simulink model "simulinkControlLoop"  (R2020b)
settings: Solver=VariableStepAuto  StartTime=0.0  StopTime=11  RelTol=1e-3
undefined symbols (not defined in the file or in its folder): DiscIntNeverNeededParam, equilibrium, K, KI, Kpend, u0jump, u0l, u0r, u3l, u3r
libraries: dspsigops x10, robotgazebolib x5, dspsrcs4 x3, robotcorelib x1
settings Model: Creator=Adam  LastModifiedBy=Adam

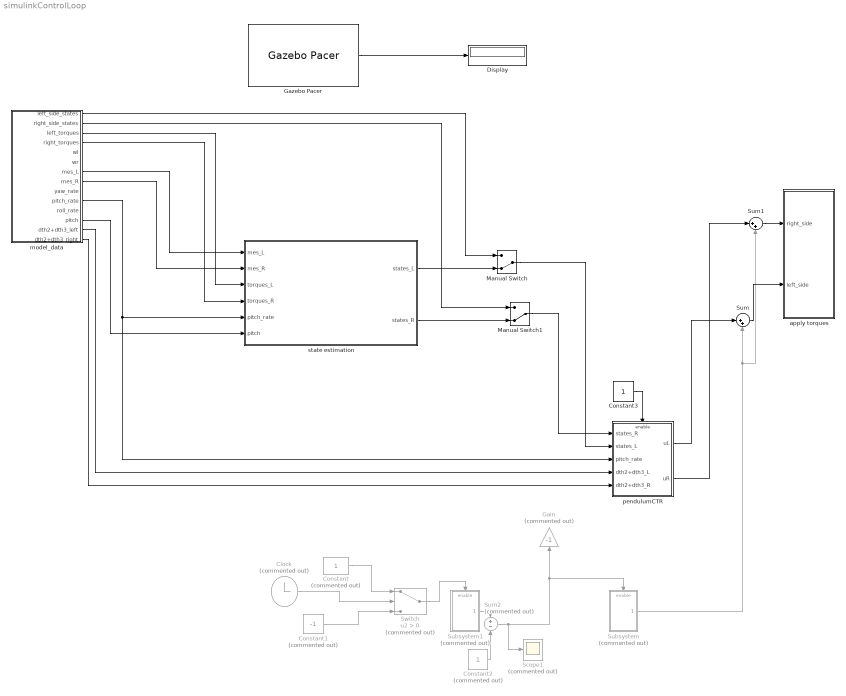
== system simulinkControlLoop ==
  Clock : Clock  Commented=on
  Constant : Constant  Commented=on
  Constant1 : Constant  Commented=on  Value=-1
  Constant2 : Constant  Commented=on
  Constant3 : Constant
  Display : Display
  Gain : Gain  Commented=on  Gain=-1
  Gazebo Pacer : robotgazebolib/Gazebo Pacer  ResetBehavior=Reset Gazebo simulation time and scene  SampleTime=0.001
      settings: SourceProductBaseCode=RO
  Manual Switch : ManualSwitch  CurrentSetting=0
  Manual Switch1 : ManualSwitch  CurrentSetting=0
  Scope1 : Scope  Commented=on
  Subsystem : Subsystem  Commented=on
  Subsystem1 : Subsystem  Commented=on
  Sum : Sum  Inputs=|++
  Sum1 : Sum  Inputs=|++
  Sum2 : Sum  Commented=on  Inputs=+-
  Switch : Switch  Commented=on  Criteria=u2 > Threshold
  apply torques : Subsystem
  model_data : Subsystem
  pendulumCTR : Subsystem
  state estimation : Subsystem
  wires:
  model_data/2(right_side_states) -> Manual Switch1/1
  Manual Switch/1 -> pendulumCTR/2(states_L)
  model_data/1(left_side_states) -> Manual Switch/1
  Manual Switch1/1 -> pendulumCTR/1(states_R)
  Gazebo Pacer/1 -> Display/1
  Constant/1 -> Switch/1
  Constant1/1 -> Switch/3
  Subsystem1/1(Output) -> Sum2/1
  Constant2/1 -> Sum2/2
  Sum2/1 -> Scope1/1, Subsystem/Enable, Gain/1
  Subsystem/1(Output) -> Sum1/2, Sum/2
  Sum1/1 -> apply torques/1(right_side)
  Sum/1 -> apply torques/2(left_side)
  pendulumCTR/1(uL) -> Sum/1
  pendulumCTR/2(uR) -> Sum1/1
  Clock/1 -> Switch/2
  Switch/1 -> Subsystem1/Enable
  Constant3/1 -> pendulumCTR/Enable
  model_data/3(left_torques) -> state estimation/3(torques_L)
  model_data/4(right_torques) -> state estimation/4(torques_R)
  state estimation/1(states_L) -> Manual Switch/2
  state estimation/2(states_R) -> Manual Switch1/2
  model_data/12(pitch) -> state estimation/6(pitch)
  model_data/7(mes_L) -> state estimation/1(mes_L)
  model_data/8(mes_R) -> state estimation/2(mes_R)
  model_data/10(pitch_rate) -> pendulumCTR/3(pitch_rate), state estimation/5(pitch_rate)
  model_data/13(dth2+dth3_left) -> pendulumCTR/4(dth2+dth3_L)
  model_data/14(dth2+dth3_right) -> pendulumCTR/5(dth2+dth3_R)

== system simulinkControlLoop/Subsystem ==
  Enable : EnablePort  StatesWhenEnabling=reset
  Mux : Mux  Inputs=2
  Signal From Workspace : dspsrcs4/Signal From Workspace  X=u3jump  Ts=0.001  nsamps=1  OutputAfterFinalValue=Setting to zero  ignoreOrWarnInputAndFrameLengths=off  OutputFrames=off
  Signal From Workspace1 : dspsrcs4/Signal From Workspace  X=u0jump  Ts=0.001  nsamps=1  OutputAfterFinalValue=Setting to zero  ignoreOrWarnInputAndFrameLengths=off  OutputFrames=off
  Output : Outport
  wires:
  Signal From Workspace1/1 -> Mux/1
  Signal From Workspace/1 -> Mux/2
  Mux/1 -> Output/1

== system simulinkControlLoop/Subsystem1 ==
  Enable : EnablePort  StatesWhenEnabling=reset
  Signal From Workspace : dspsrcs4/Signal From Workspace  X=2*ones(numel(u0jump),1)  Ts=0.001  nsamps=1  OutputAfterFinalValue=Setting to zero  ignoreOrWarnInputAndFrameLengths=off  OutputFrames=off
  Output : Outport
  wires:
  Signal From Workspace/1 -> Output/1

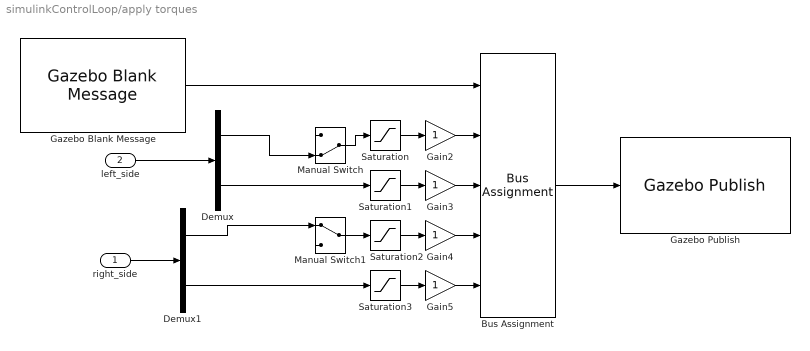
== system simulinkControlLoop/apply torques ==
  right_side : Inport
  left_side : Inport  Port=2
  Bus Assignment : BusAssignment  AssignedSignals=u0l,u3l,u0r,u3r
  Demux : Demux  Outputs=2
  Demux1 : Demux  Outputs=2
  Gain{2..5} (4 alike) : Gain
  Gazebo Blank Message : robotgazebolib/Gazebo Blank Message  msgType=gazebo_msgs/custom/19XzAhyZzP/Contro1XtejReiyv  sampleTime=0.001  busName='Gazebo_SL_Bus_gazebo_msgs_custom_19XzAhyZzP_Contro1XtejReiyv'
      settings: SourceProductBaseCode=RO
  Gazebo Publish : robotgazebolib/Gazebo Publish  topicSource=Specify your own  topic=/gazebo/default/controlCommand  messageType=gazebo_msgs/custom/19XzAhyZzP/Contro1XtejReiyv  sampleTime=0.001
      settings: SourceProductBaseCode=RO
  Manual Switch : ManualSwitch  CurrentSetting=0
  Manual Switch1 : ManualSwitch
  Saturation : Saturate  UpperLimit=2  LowerLimit=-2
  Saturation1 : Saturate  UpperLimit=10  LowerLimit=-10
  Saturation2 : Saturate  UpperLimit=2  LowerLimit=-2
  Saturation3 : Saturate  UpperLimit=10  LowerLimit=-10
  wires:
  Gain3/1 -> Bus Assignment/3
  Saturation3/1 -> Gain5/1
  Saturation/1 -> Gain2/1
  Demux/2 -> Saturation1/1
  Bus Assignment/1 -> Gazebo Publish/1
  Saturation1/1 -> Gain3/1
  Demux1/2 -> Saturation3/1
  Gazebo Blank Message/1 -> Bus Assignment/1
  Gain5/1 -> Bus Assignment/5
  Saturation2/1 -> Gain4/1
  left_side/1 -> Demux/1
  right_side/1 -> Demux1/1
  Demux1/1 -> Manual Switch1/1
  Demux/1 -> Manual Switch/2
  Gain2/1 -> Bus Assignment/2
  Gain4/1 -> Bus Assignment/4
  Manual Switch/1 -> Saturation/1
  Manual Switch1/1 -> Saturation2/1

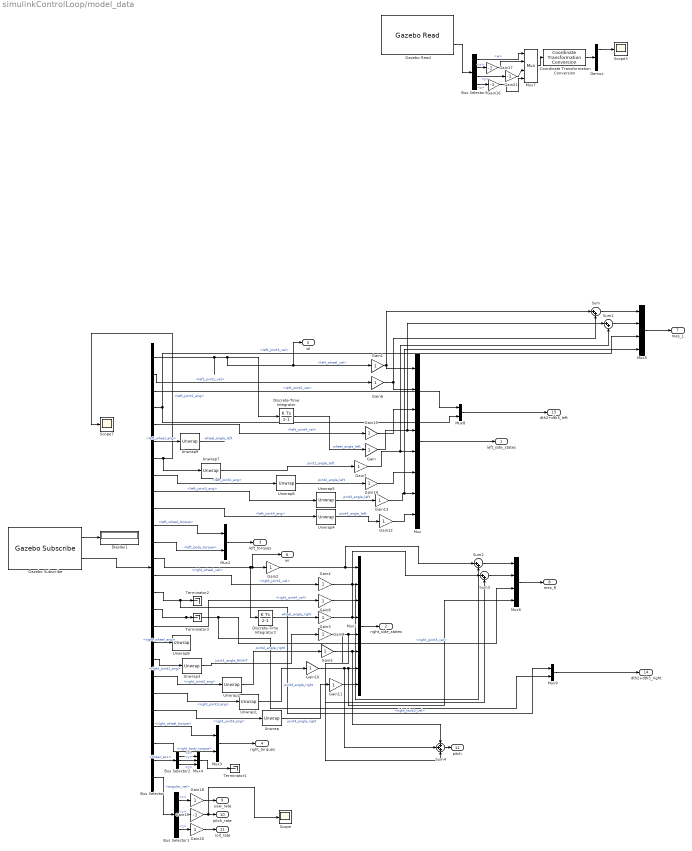
== system simulinkControlLoop/model_data ==
  Bus Selector : BusSelector  OutputSignals=left_wheel_vel,left_joint1_vel,left_joint2_vel,left_joint3_vel,left_joint4_vel,left_wheel_ang,left_joint1_ang,left_joint2_ang,left_joint3_ang,left_joint4_ang,left_wheel_torque,left_body_torque,right_wheel_vel,right_joint1_vel,right_joint2_vel,right_joint3_vel,right_joint4_vel,right_wheel_ang,right_joint1_ang,right_joint2_ang,right_joint3_ang,right_joint4_ang,right_wheel_torque,right_body_torque,linear_acc,angular_vel
  Bus Selector1 : BusSelector  OutputSignals=x,y,z
  Bus Selector2 : BusSelector  OutputSignals=x,y,z
  Bus Selector3 : BusSelector  OutputSignals=world_pose.orientation.w,world_pose.orientation.x,world_pose.orientation.y,world_pose.orientation.z
  Coordinate Transformation Conversion : robotcorelib/Coordinate Transformation Conversion  InputRepresentation=Quaternion  InputEulerSequence=ZYX  ShowTrVecInputPort=on  OutputRepresentation=Euler Angles  OutputEulerSequence=ZYX  ShowTrVecOutputPort=on  SimulateUsing=Interpreted execution
  Demux : Demux  Outputs=3
  Discrete-Time Integrator : DiscreteIntegrator  gainval=1  SampleTime=-1  ICPrevOutput=DiscIntNeverNeededParam  ICPrevScaledInput=DiscIntNeverNeededParam
  Discrete-Time Integrator2 : DiscreteIntegrator  gainval=1  SampleTime=-1  ICPrevOutput=DiscIntNeverNeededParam  ICPrevScaledInput=DiscIntNeverNeededParam
  Display1 : Display
  Gain{,1..15,18,20} (18 alike) : Gain
  Gain{16..17,19,21} (4 alike) : Gain  Gain=-1
  Gazebo Read : robotgazebolib/Gazebo Read  topicSource=From Gazebo  topic=/gazebo/ground_truth/link_state/Stoupento/Stoupento::left_wheel  messageType=gazebo_msgs/LinkState  sampleTime=0.001
      settings: SourceProductBaseCode=RO
  Gazebo Subscribe : robotgazebolib/Gazebo Subscribe  topicSource=From Gazebo  topic=/gazebo/default/stoupentoMesurement  messageType=gazebo_msgs/custom/19XzAhyZzP/Stoupe1grC5VeUzD  sampleTime=0.001
      settings: SourceProductBaseCode=RO
  Mux : Mux  Inputs=8
  Mux1 : Mux  Inputs=8
  Mux{2..3,8..9} (4 alike) : Mux  Inputs=2
  Mux4 : Mux  Inputs=3
  Mux5 : Mux
  Mux6 : Mux
  Mux7 : Mux
  Scope : Scope
  Scope3 : Scope
  Scope7 : Scope
  Sum{,1..3} (4 alike) : Sum  Inputs=|++
  Sum4 : Sum  Inputs=+++
  Terminator1 : Terminator
  Terminator2 : Terminator
  Terminator3 : Terminator
  Unwrap{,1..2,4..6} (6 alike) : dspsigops/Unwrap  tol=pi  InputProcessing=Columns as channels (frame based)  running=off
  Unwrap3 : dspsigops/Unwrap  tol=19/10*pi  InputProcessing=Columns as channels (frame based)  running=off
  Unwrap7 : dspsigops/Unwrap  tol=19/10*pi  InputProcessing=Columns as channels (frame based)  running=off
  Unwrap8 : dspsigops/Unwrap  tol=19*pi/10  InputProcessing=Columns as channels (frame based)  running=off
  Unwrap9 : dspsigops/Unwrap  tol=19/10*pi  InputProcessing=Columns as channels (frame based)  running=off
  left_side_states : Outport
  right_side_states : Outport  Port=2
  left_torques : Outport  Port=3
  right_torques : Outport  Port=4
  wl : Outport  Port=5
  wr : Outport  Port=6
  mes_L : Outport  Port=7
  mes_R : Outport  Port=8
  yaw_rate : Outport  Port=9
  pitch_rate : Outport  Port=10
  roll_rate : Outport  Port=11
  pitch : Outport  Port=12
  dth2+dth3_left : Outport  Port=13
  dth2+dth3_right : Outport  Port=14
  wires:
  Gazebo Subscribe/1 -> Display1/1
  Bus Selector/23 -> Mux3/1  "<right_wheel_torque>"
  Bus Selector/12 -> Mux2/2  "<left_body_torque>"
  Bus Selector/18 -> Unwrap8/1  "<right_wheel_ang>"
  Bus Selector/5 -> Gain15/1  "<left_joint4_vel>"
  Bus Selector/9 -> Unwrap5/1  "<left_joint3_ang>"
  Bus Selector/20 -> Unwrap2/1  "<right_joint2_ang>"
  Bus Selector/22 -> Unwrap/1  "<right_joint4_ang>"
  Bus Selector/8 -> Unwrap6/1  "<left_joint2_ang>"
  Unwrap1/1 -> Gain10/1  "joint3_angle_right"
  Unwrap/1 -> Gain11/1  "joint4_angle_right"
  Unwrap4/1 -> Gain12/1  "joint4_angle_left"
  Gazebo Subscribe/2 -> Bus Selector/1
  Bus Selector/19 -> Unwrap3/1  "<right_joint1_ang>"
  Bus Selector/6 -> Unwrap9/1  "<left_wheel_ang>"
  Unwrap5/1 -> Gain13/1  "joint3_angle_left"
  Bus Selector/7 -> Unwrap7/1, Scope7/1  "<left_joint1_ang>"
  Bus Selector/10 -> Unwrap4/1  "<left_joint4_ang>"
  Unwrap6/1 -> Gain14/1  "joint2_angle_left"
  Bus Selector/21 -> Unwrap1/1  "<right_joint3_ang>"
  Unwrap9/1 -> ?  "wheel_angle_left"
  Mux/1 -> left_side_states/1
  Bus Selector/24 -> Mux3/2  "<right_body_torque>"
  Bus Selector/3 -> Mux8/1  "<left_joint2_vel>"
  Bus Selector/11 -> Mux2/1  "<left_wheel_torque>"
  Mux2/1 -> left_torques/1
  Mux3/1 -> right_torques/1
  Bus Selector/17 -> Gain8/1  "<right_joint4_vel>"
  Bus Selector/13 -> Discrete-Time Integrator2/1, wr/1, Gain2/1  "<right_wheel_vel>"
  Unwrap2/1 -> Gain5/1  "joint2_angle_right"
  Mux1/1 -> right_side_states/1
  Gain3/1 -> Sum3/1, Mux1/4
  Gain4/1 -> Sum2/2, Mux1/2
  Gain5/1 -> Sum4/1, Mux1/6
  Gain8/1 -> Mux1/3
  Gain11/1 -> Mux1/8
  Bus Selector/25 -> Bus Selector2/1  "<linear_acc>"
  Bus Selector/4 -> Mux5/3, Mux8/2  "<left_joint3_vel>"
  Bus Selector/26 -> Bus Selector1/1  "<angular_vel>"
  Gain10/1 -> Sum4/2, Mux6/4, Mux1/7
  Bus Selector2/1 -> Mux4/1  "<x>"
  Bus Selector2/2 -> Mux4/2  "<y>"
  Bus Selector2/3 -> Mux4/3  "<z>"
  Gain2/1 -> Sum2/1, Mux1/1
  Bus Selector/1 -> Discrete-Time Integrator/1, Gain1/1, wl/1  "<left_wheel_vel>"
  Gain1/1 -> Sum/1, Mux/1
  Gain6/1 -> Sum/2, Mux/2
  Mux5/1 -> mes_L/1
  Mux6/1 -> mes_R/1
  Mux4/1 -> Terminator1/1
  Bus Selector1/1 -> Gain18/1  "<x>"
  Bus Selector1/2 -> Gain19/1  "<y>"
  Bus Selector1/3 -> Gain20/1  "<z>"
  Gain18/1 -> yaw_rate/1
  Gain19/1 -> Scope/1, pitch_rate/1
  Gain20/1 -> roll_rate/1
  Gazebo Read/2 -> Bus Selector3/1
  Bus Selector3/1 -> Mux7/1  "<w>"
  Bus Selector3/2 -> Gain17/1  "<x>"
  Bus Selector3/3 -> Gain21/1  "<y>"
  Bus Selector3/4 -> Gain16/1  "<z>"
  Mux7/1 -> Coordinate Transformation Conversion/1
  Coordinate Transformation Conversion/1 -> Demux/1
  Gain16/1 -> Mux7/4
  Gain21/1 -> Mux7/3
  Gain17/1 -> Mux7/2
  Demux/1 -> Scope3/1
  Discrete-Time Integrator/1 -> Gain/1  "wheel_angle_left"
  Discrete-Time Integrator2/1 -> Gain3/1  "wheel_angle_right"
  Bus Selector/2 -> Gain6/1  "<left_joint1_vel>"
  Bus Selector/14 -> Gain4/1  "<right_joint1_vel>"
  Unwrap3/1 -> Gain9/1  "joint1_angle_RIGHT"
  Unwrap7/1 -> Gain7/1  "joint1_angle_left"
  Sum/1 -> Mux5/1
  Sum1/1 -> Mux5/2
  Sum2/1 -> Mux6/1
  Sum3/1 -> Mux6/2
  Gain9/1 -> Sum3/2, Sum4/3, Mux1/5
  Sum4/1 -> pitch/1
  Gain15/1 -> Mux/3
  Gain/1 -> Sum1/1, Mux/4
  Gain7/1 -> Sum1/2, Mux/5
  Gain14/1 -> Mux/6
  Gain13/1 -> Mux5/4, Mux/7
  Gain12/1 -> Mux/8
  Mux8/1 -> dth2+dth3_left/1
  Bus Selector/16 -> Mux9/2, Mux6/3, Terminator3/1  "<right_joint3_vel>"
  Mux9/1 -> dth2+dth3_right/1
  Bus Selector/15 -> Mux9/1, Terminator2/1  "<right_joint2_vel>"

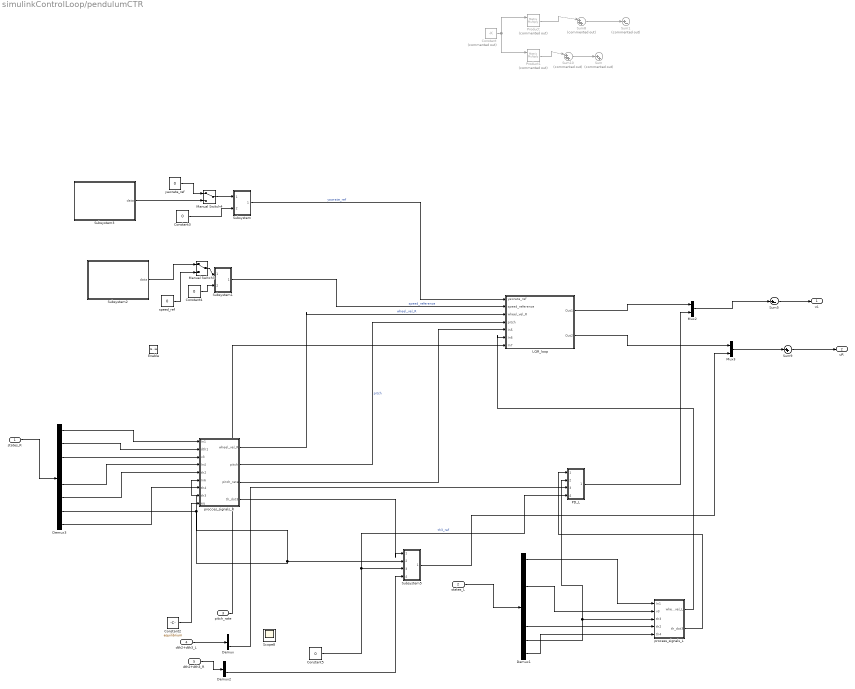
== system simulinkControlLoop/pendulumCTR ==
  states_R : Inport
  states_L : Inport  Port=2
  pitch_rate : Inport  Port=3
  dth2+dth3_L : Inport  Port=4
  dth2+dth3_R : Inport  Port=5
  Enable : EnablePort  StatesWhenEnabling=reset
  Constant : Constant  Commented=on  Value=-K
  Constant2 : Constant  Value=equilibrium
  Constant3 : Constant  Value=0
  Constant4 : Constant  Value=0
  Constant5 : Constant  Value=0
  Demux : Demux  Outputs=2
  Demux1 : Demux  Outputs=8
  Demux2 : Demux  Outputs=2
  Demux3 : Demux  Outputs=8
  LQR_loop : Subsystem
  Manual Switch3 : ManualSwitch
  Manual Switch4 : ManualSwitch
  Mux2 : Mux  Inputs=2
  Mux3 : Mux  Inputs=3
  PD_L : Subsystem
  Product : Product  Commented=on  Multiplication=Matrix(*)
  Product1 : Product  Commented=on  Multiplication=Matrix(*)
  Scope8 : Scope  NumInputPorts=2
  Subsystem : Subsystem
  Subsystem1 : Subsystem
  Subsystem2 : Subsystem
  Subsystem3 : Subsystem
  Subsystem5 : Subsystem
  Sum : Sum  Commented=on  Inputs=|++
  Sum1 : Sum  Commented=on  Inputs=|+-
  Sum10 : Sum  Commented=on  Inputs=|+++
  Sum5 : Sum  Inputs=|+-
  Sum8 : Sum  Commented=on  Inputs=|+++
  Sum9 : Sum  Inputs=|++
  procces_signals_R : Subsystem
  process_signals_L : Subsystem
  speed_ref : Constant  Value=0  SampleTime=0.001
  yawrate_ref : Constant  Value=0  SampleTime=0.001
  uL : Outport
  uR : Outport  Port=2
  wires:
  Constant/1 -> Product/1, Product1/1
  Product/1 -> Sum8/1
  Sum8/1 -> Sum1/1
  Product1/1 -> Sum10/1
  Sum10/1 -> Sum/1
  states_R/1 -> Demux3/1
  states_L/1 -> Demux1/1
  Demux3/7 -> procces_signals_R/8(th3), Subsystem5/2(In2), procces_signals_R/6(In6)
  Sum5/1 -> uL/1
  Mux2/1 -> Sum5/1
  Sum9/1 -> uR/1
  Mux3/1 -> Sum9/1
  Constant3/1 -> Subsystem/2(lambda)
  Constant4/1 -> Subsystem1/2(lambda)
  Constant5/1 -> PD_L/4(th3_ref), Subsystem5/3(th3_ref)  "th3_ref"
  Demux1/7 -> process_signals_L/3(th3), PD_L/2(In2)
  dth2+dth3_L/1 -> Demux/1
  dth2+dth3_R/1 -> Demux2/1
  Subsystem2/1(data) -> Manual Switch3/1
  Manual Switch4/1 -> Subsystem/1(data)
  Subsystem3/1(data) -> Manual Switch4/2
  yawrate_ref/1 -> Manual Switch4/1
  Manual Switch3/1 -> Subsystem1/1(data)
  speed_ref/1 -> Manual Switch3/2
  Demux3/1 -> procces_signals_R/1(In1)
  Demux3/2 -> procces_signals_R/2(dth1)
  Demux3/3 -> procces_signals_R/3(v3)
  Demux3/5 -> procces_signals_R/4(In4)
  Demux3/6 -> procces_signals_R/5(th2)
  Demux3/8 -> procces_signals_R/7(th4)
  Constant2/1 -> procces_signals_R/9(eq)
  procces_signals_R/4(th_dot3) -> Subsystem5/1(In1)
  Demux2/2 -> Subsystem5/4(In4)
  Subsystem5/1(Out1) -> Mux3/3
  Demux/2 -> PD_L/3(In3)
  PD_L/1(Out1) -> Mux2/2
  Demux1/1 -> process_signals_L/1(In1)
  Demux1/3 -> process_signals_L/2(v3)
  Demux1/6 -> process_signals_L/4(th2)
  Demux1/8 -> process_signals_L/5(th4)
  process_signals_L/2(th_dot3) -> PD_L/1(In1)
  Subsystem/1(Out1) -> LQR_loop/1(yawrate_ref)  "yawrate_ref"
  Subsystem1/1(Out1) -> LQR_loop/2(speed_reference)  "speed_reference"
  procces_signals_R/1(wheel_vel_R) -> LQR_loop/3(wheel_vel_R)  "wheel_vel_R"
  procces_signals_R/2(pitch) -> LQR_loop/4(pitch)  "pitch"
  procces_signals_R/3(pitch_rate) -> LQR_loop/5(In5)
  process_signals_L/1(wheel_vel_L) -> LQR_loop/6(In6)
  pitch_rate/1 -> LQR_loop/7(In7)
  LQR_loop/1(Out1) -> Mux2/1
  LQR_loop/2(Out2) -> Mux3/1

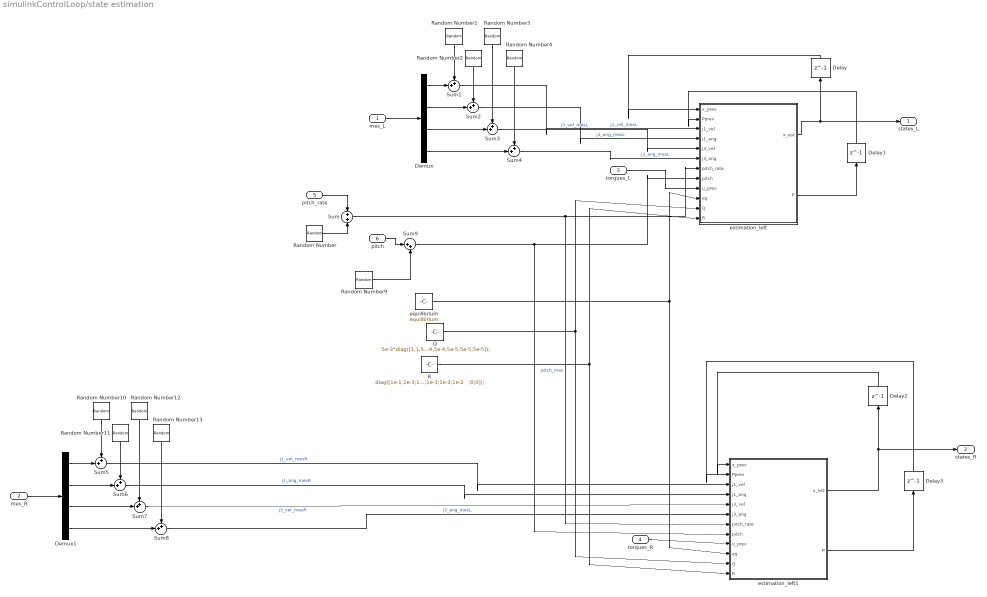
== system simulinkControlLoop/state estimation ==
  mes_L : Inport
  mes_R : Inport  Port=2
  torques_L : Inport  Port=3
  torques_R : Inport  Port=4
  pitch_rate : Inport  Port=5
  pitch : Inport  Port=6
  Delay : Delay  DelayLength=1  InitialCondition=[0;0;0;0;0;0;0;0]  SampleTime=0.001
  Delay1 : Delay  DelayLength=1  InitialCondition=1e-6*eye(8)  SampleTime=0.001
  Delay2 : Delay  DelayLength=1  InitialCondition=[0;0;0;0;0;0;0;0]  SampleTime=0.001
  Delay3 : Delay  DelayLength=1  InitialCondition=1e-6*eye(8)  SampleTime=0.001
  Demux : Demux
  Demux1 : Demux
  Q : Constant  Value=5e-3*diag([1,1,5e-2,5e-4,5e-4,5e-5,5e-5,5e-5]);
  R : Constant  Value="diag([1e-1;1e-3;1e-1;1e-3;1e-2;1e-2   ;0;0]);"
  Random Number : RandomNumber  Variance=1e-2  Seed=randi([0 100])  SampleTime=0.001
  Random Number{1,3,10,12} (4 alike) : RandomNumber  Variance=1e-1  Seed=randi([0 100])  SampleTime=0.001
  Random Number{2,4,11,13} (4 alike) : RandomNumber  Variance=1e-3  Seed=randi([0 100])  SampleTime=0.001
  Random Number9 : RandomNumber  Variance=1e-2  Seed=randi([0 100])  SampleTime=0.001
  Sum : Sum
  Sum{1..8} (8 alike) : Sum  Inputs=++|
  Sum9 : Sum  Inputs=|++
  equilibrium : Constant  Value=equilibrium
  estimation_left : MATLAB Function  TreatAsAtomicUnit=on
  estimation_left1 : MATLAB Function  TreatAsAtomicUnit=on
  states_L : Outport
  states_R : Outport  Port=2
  wires:
  torques_L/1 -> estimation_left/9(u_prev)
  estimation_left/1(x_est) -> states_L/1, Delay/1
  Delay/1 -> estimation_left/1(x_prev)
  estimation_left/2(P) -> Delay1/1
  Delay1/1 -> estimation_left/2(Pprev)
  pitch_rate/1 -> Sum/1
  Random Number/1 -> Sum/2
  mes_L/1 -> Demux/1
  Demux/1 -> Sum1/2
  Demux/2 -> Sum2/2
  Demux/3 -> Sum3/2
  Demux/4 -> Sum4/2
  Random Number4/1 -> Sum4/1
  Random Number3/1 -> Sum3/1
  Random Number2/1 -> Sum2/1
  Random Number1/1 -> Sum1/1
  Sum1/1 -> estimation_left/3(j1_vel)  "j1_vel_mesL"
  Sum2/1 -> estimation_left/4(j1_ang)  "j1_ang_mesL"
  Sum3/1 -> estimation_left/5(j3_vel)  "j3_vel_mesL"
  Sum4/1 -> estimation_left/6(j3_ang)  "j3_ang_mesL"
  R/1 -> estimation_left1/12(R), estimation_left/12(R)
  Sum/1 -> estimation_left1/7(pitch_rate), estimation_left/7(pitch_rate)  "pitch_mes"
  Sum5/1 -> estimation_left1/3(j1_vel)  "j1_vel_mesR"
  Sum8/1 -> estimation_left1/6(j3_ang)  "j3_ang_mesL"
  Sum6/1 -> estimation_left1/4(j1_ang)  "j1_ang_mesR"
  Random Number13/1 -> Sum8/1
  Random Number11/1 -> Sum6/1
  equilibrium/1 -> estimation_left1/10(eq), estimation_left/10(eq)
  Demux1/4 -> Sum8/2
  Q/1 -> estimation_left/11(Q), estimation_left1/11(Q)
  Sum7/1 -> estimation_left1/5(j3_vel)  "j3_vel_mesR"
  Demux1/2 -> Sum6/2
  torques_R/1 -> estimation_left1/9(u_prev)
  mes_R/1 -> Demux1/1
  Demux1/3 -> Sum7/2
  Demux1/1 -> Sum5/2
  pitch/1 -> Sum9/1
  Random Number9/1 -> Sum9/2
  Sum9/1 -> estimation_left1/8(pitch), estimation_left/8(pitch)
  Random Number10/1 -> Sum5/1
  Random Number12/1 -> Sum7/1
  estimation_left1/2(P) -> Delay3/1
  Delay2/1 -> estimation_left1/1(x_prev)
  estimation_left1/1(x_est) -> states_R/1, Delay2/1
  Delay3/1 -> estimation_left1/2(Pprev)

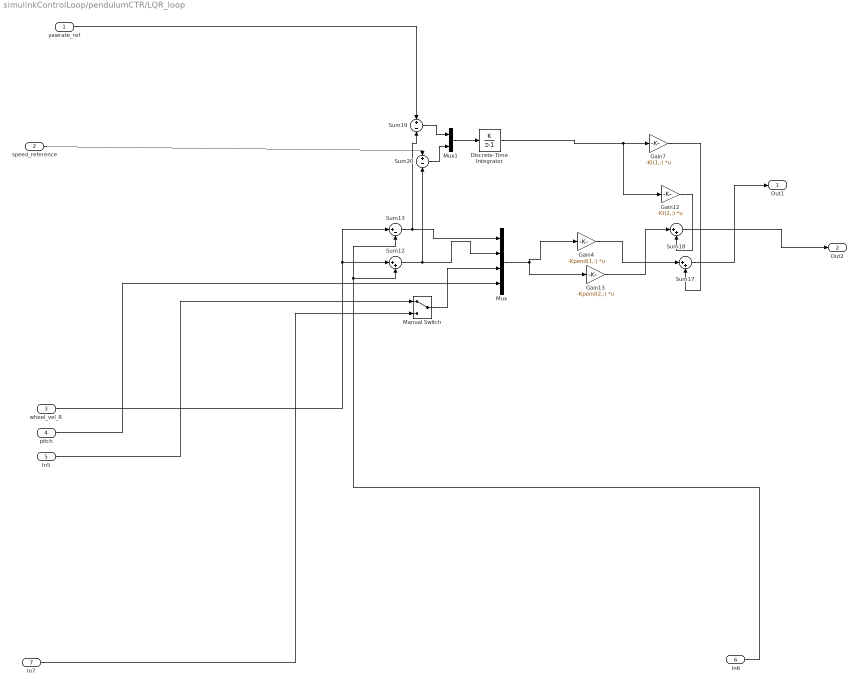
== system simulinkControlLoop/pendulumCTR/LQR_loop ==
  yawrate_ref : Inport
  speed_reference : Inport  Port=2
  wheel_vel_R : Inport  Port=3
  pitch : Inport  Port=4
  In5 : Inport  Port=5
  In6 : Inport  Port=6
  In7 : Inport  Port=7
  Discrete-Time Integrator : DiscreteIntegrator  IntegratorMethod=Accumulation: Forward Euler  gainval=1  SampleTime=0.001  ICPrevOutput=DiscIntNeverNeededParam  ICPrevScaledInput=DiscIntNeverNeededParam
  Gain12 : Gain  Gain=-KI(2,:)  Multiplication=Matrix(K*u)
  Gain13 : Gain  Gain=-Kpend(2,:)  Multiplication=Matrix(K*u)
  Gain4 : Gain  Gain=-Kpend(1,:)  Multiplication=Matrix(K*u)
  Gain7 : Gain  Gain=-KI(1,:)  Multiplication=Matrix(K*u)
  Manual Switch : ManualSwitch
  Mux : Mux
  Mux1 : Mux  Inputs=2
  Sum12 : Sum  Inputs=|++
  Sum13 : Sum  Inputs=|+-
  Sum17 : Sum  Inputs=|++
  Sum18 : Sum  Inputs=|++
  Sum19 : Sum  Inputs=+-
  Sum20 : Sum  Inputs=+-
  Out1 : Outport
  Out2 : Outport  Port=2
  wires:
  Discrete-Time Integrator/1 -> Gain12/1, Gain7/1
  wheel_vel_R/1 -> Sum13/1, Sum12/1
  Sum13/1 -> Sum19/2, Mux/1
  yawrate_ref/1 -> Sum19/1
  Sum19/1 -> Mux1/1
  Sum12/1 -> Sum20/2, Mux/2
  Mux/1 -> Gain4/1, Gain13/1
  In6/1 -> Sum12/2, Sum13/2
  Gain12/1 -> Sum18/2
  Gain4/1 -> Sum17/1
  Mux1/1 -> Discrete-Time Integrator/1
  Sum20/1 -> Mux1/2
  pitch/1 -> Mux/4
  Manual Switch/1 -> Mux/3
  Gain13/1 -> Sum18/1
  Gain7/1 -> Sum17/2
  Sum17/1 -> Out1/1
  Sum18/1 -> Out2/1
  In7/1 -> Manual Switch/2
  speed_reference/1 -> Sum20/1
  In5/1 -> Manual Switch/1

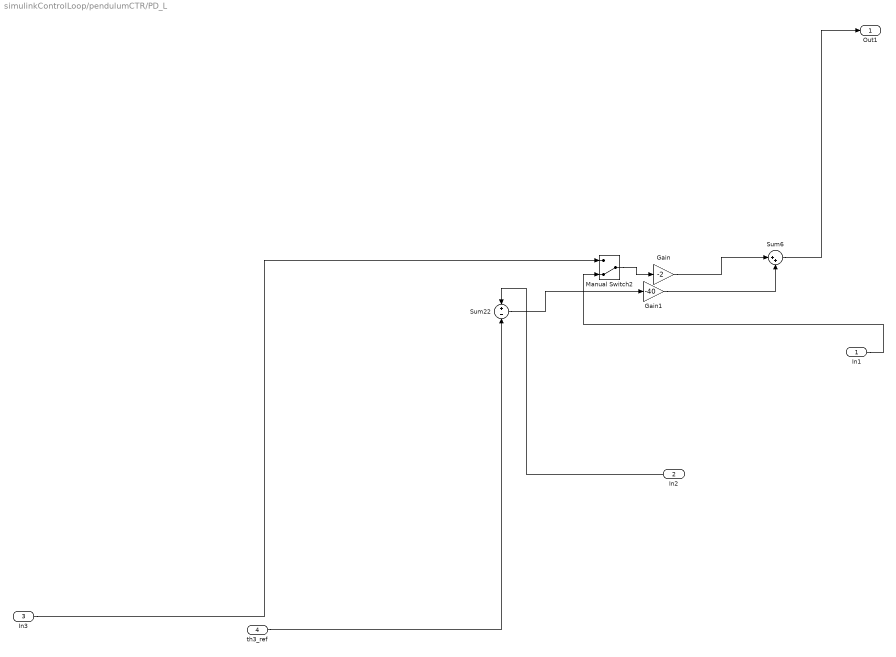
== system simulinkControlLoop/pendulumCTR/PD_L ==
  In1 : Inport
  In2 : Inport  Port=2
  In3 : Inport  Port=3
  th3_ref : Inport  Port=4
  Gain : Gain  Gain=-2
  Gain1 : Gain  Gain=-40
  Manual Switch2 : ManualSwitch  CurrentSetting=0
  Sum22 : Sum  Inputs=+-
  Sum6 : Sum  Inputs=|++
  Out1 : Outport
  wires:
  In3/1 -> Manual Switch2/1
  In2/1 -> Sum22/1
  th3_ref/1 -> Sum22/2
  Gain1/1 -> Sum6/2
  Gain/1 -> Sum6/1
  Sum22/1 -> Gain1/1
  Sum6/1 -> Out1/1
  In1/1 -> Manual Switch2/2
  Manual Switch2/1 -> Gain/1

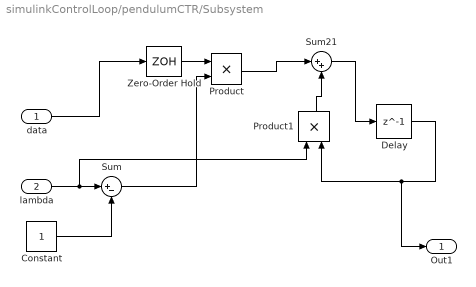
== system simulinkControlLoop/pendulumCTR/Subsystem ==
  data : Inport
  lambda : Inport  Port=2
  Constant : Constant
  Delay : Delay  DelayLength=1  SampleTime=0.01
  Product : Product
  Product1 : Product
  Sum : Sum  Inputs=|+-
  Sum21 : Sum  Inputs=|++
  Zero-Order Hold : ZeroOrderHold  SampleTime=0.01
  Out1 : Outport
  wires:
  Sum21/1 -> Delay/1
  Delay/1 -> Product1/2, Out1/1
  Product/1 -> Sum21/1
  Zero-Order Hold/1 -> Product/1
  lambda/1 -> Product1/1, Sum/1
  Constant/1 -> Sum/2
  Sum/1 -> Product/2
  Product1/1 -> Sum21/2
  data/1 -> Zero-Order Hold/1

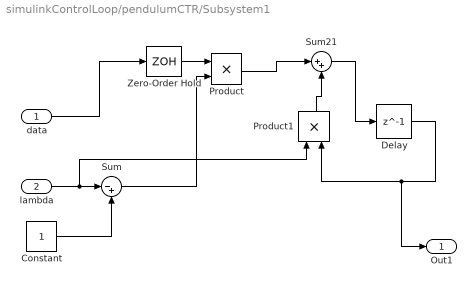
== system simulinkControlLoop/pendulumCTR/Subsystem1 ==
  data : Inport
  lambda : Inport  Port=2
  Constant : Constant
  Delay : Delay  DelayLength=1  SampleTime=0.01
  Product : Product
  Product1 : Product
  Sum : Sum  Inputs=|-+
  Sum21 : Sum  Inputs=|++
  Zero-Order Hold : ZeroOrderHold  SampleTime=0.01
  Out1 : Outport
  wires:
  Sum21/1 -> Delay/1
  Delay/1 -> Product1/2, Out1/1
  Product/1 -> Sum21/1
  Zero-Order Hold/1 -> Product/1
  lambda/1 -> Product1/1, Sum/1
  Constant/1 -> Sum/2
  Sum/1 -> Product/2
  Product1/1 -> Sum21/2
  data/1 -> Zero-Order Hold/1

== system simulinkControlLoop/pendulumCTR/Subsystem2 ==
  Step : Step  Time=2  After=-15  SampleTime=0
  Step1 : Step  Time=7.5  After=15  SampleTime=0
  Sum : Sum  Inputs=|++
  data : Outport
  wires:
  Step/1 -> Sum/1
  Step1/1 -> Sum/2
  Sum/1 -> data/1

== system simulinkControlLoop/pendulumCTR/Subsystem3 ==
  Step : Step  Time=4.5  After=5  SampleTime=0
  Step1 : Step  Time=7.5  After=-5  SampleTime=0
  Sum : Sum  Inputs=|++
  data : Outport
  wires:
  Step/1 -> Sum/1
  Step1/1 -> Sum/2
  Sum/1 -> data/1

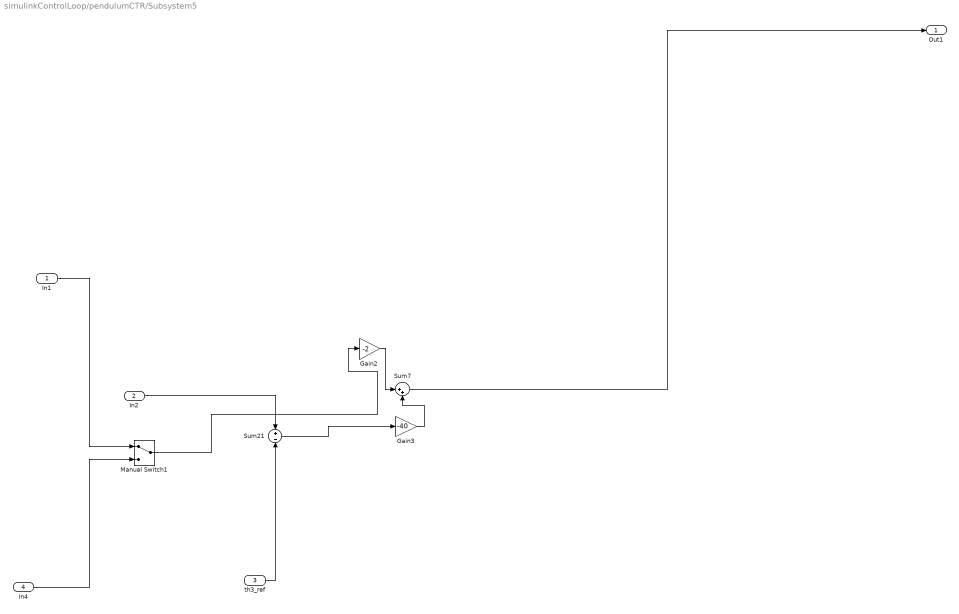
== system simulinkControlLoop/pendulumCTR/Subsystem5 ==
  In1 : Inport
  In2 : Inport  Port=2
  th3_ref : Inport  Port=3
  In4 : Inport  Port=4
  Gain2 : Gain  Gain=-2
  Gain3 : Gain  Gain=-40
  Manual Switch1 : ManualSwitch
  Sum21 : Sum  Inputs=+-
  Sum7 : Sum  Inputs=|++
  Out1 : Outport
  wires:
  In4/1 -> Manual Switch1/2
  Gain3/1 -> Sum7/2
  In2/1 -> Sum21/1
  Gain2/1 -> Sum7/1
  Sum21/1 -> Gain3/1
  th3_ref/1 -> Sum21/2
  Manual Switch1/1 -> Gain2/1
  In1/1 -> Manual Switch1/1
  Sum7/1 -> Out1/1

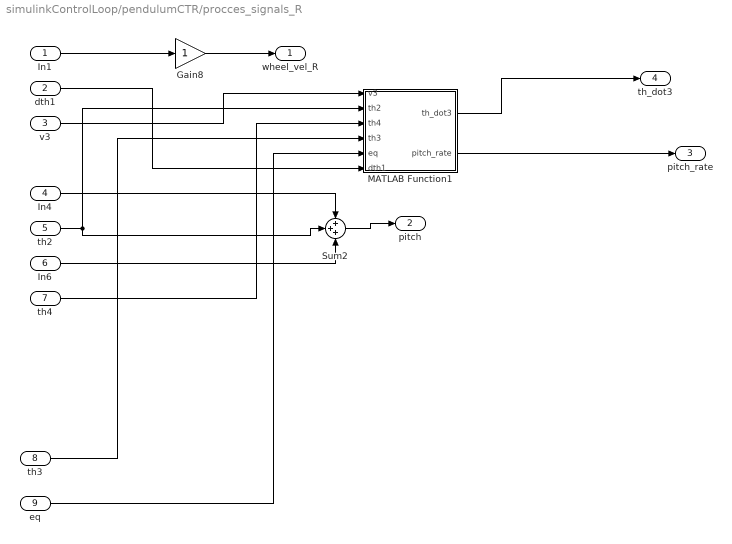
== system simulinkControlLoop/pendulumCTR/procces_signals_R ==
  In1 : Inport
  dth1 : Inport  Port=2
  v3 : Inport  Port=3
  In4 : Inport  Port=4
  th2 : Inport  Port=5
  In6 : Inport  Port=6
  th4 : Inport  Port=7
  th3 : Inport  Port=8
  eq : Inport  Port=9
  Gain8 : Gain
  MATLAB Function1 : MATLAB Function  TreatAsAtomicUnit=on
  Sum2 : Sum  Inputs=+++
  wheel_vel_R : Outport
  pitch : Outport  Port=2
  pitch_rate : Outport  Port=3
  th_dot3 : Outport  Port=4
  wires:
  th2/1 -> Sum2/2, MATLAB Function1/2(th2)
  Sum2/1 -> pitch/1
  In4/1 -> Sum2/1
  v3/1 -> MATLAB Function1/1(v3)
  th3/1 -> MATLAB Function1/4(th3)
  MATLAB Function1/1(th_dot3) -> th_dot3/1
  eq/1 -> MATLAB Function1/5(eq)
  In6/1 -> Sum2/3
  Gain8/1 -> wheel_vel_R/1
  dth1/1 -> MATLAB Function1/6(dth1)
  In1/1 -> Gain8/1
  MATLAB Function1/2(pitch_rate) -> pitch_rate/1
  th4/1 -> MATLAB Function1/3(th4)

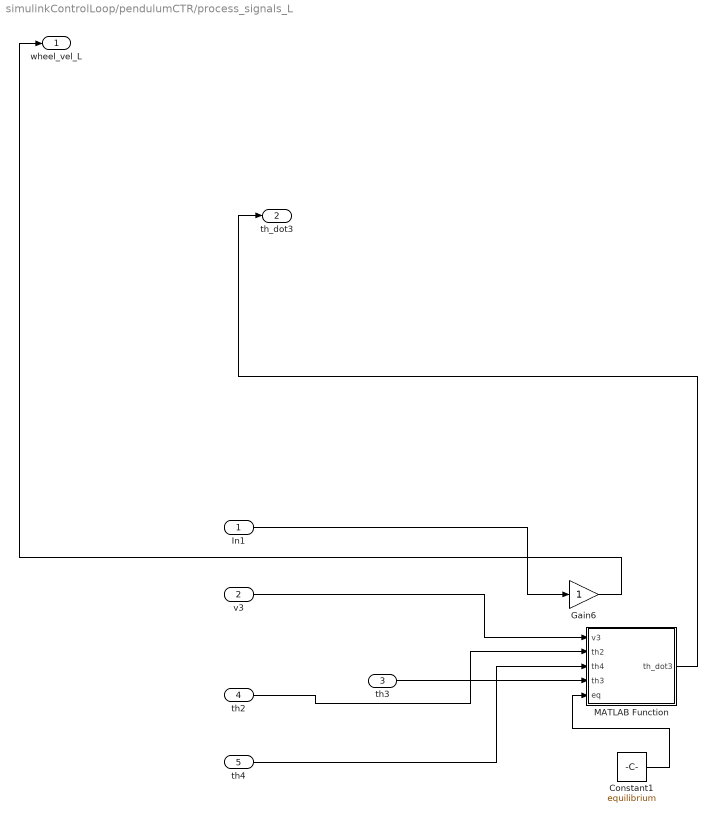
== system simulinkControlLoop/pendulumCTR/process_signals_L ==
  In1 : Inport
  v3 : Inport  Port=2
  th3 : Inport  Port=3
  th2 : Inport  Port=4
  th4 : Inport  Port=5
  Constant1 : Constant  Value=equilibrium
  Gain6 : Gain
  MATLAB Function : MATLAB Function  TreatAsAtomicUnit=on
  wheel_vel_L : Outport
  th_dot3 : Outport  Port=2
  wires:
  Constant1/1 -> MATLAB Function/5(eq)
  v3/1 -> MATLAB Function/1(v3)
  th2/1 -> MATLAB Function/2(th2)
  In1/1 -> Gain6/1
  th4/1 -> MATLAB Function/3(th4)
  Gain6/1 -> wheel_vel_L/1
  th3/1 -> MATLAB Function/4(th3)
  MATLAB Function/1(th_dot3) -> th_dot3/1

== matlab function simulinkControlLoop/state estimation/estimation_left1 ==
  data: x_prev input; x_est output; Pprev input; j1_vel input; j1_ang input; j3_vel input; j3_ang input; pitch_rate input; pitch input; u_prev input; eq input; P output; Q input; R input
function [x_est,P] = fcn(x_prev,Pprev,j1_vel,j1_ang,j3_vel,j3_ang,pitch_rate,pitch,u_prev,eq,Q,R)

x_est = zeros(8,1);
P = zeros(8,8);
k_spring = eq(5);
kang = eq(6);
nx = 8;
alpha = 1e-3;
kappa = 0;
beta = 2;
lambda = alpha^2*(nx+kappa);
weights = zeros(2*nx+1,1);
weights(1) = (lambda/(nx+lambda));
weights(2:end) = (1/(2*(nx+lambda))); 


weightsP = zeros(2*nx+1,1);
weightsP(1) = (lambda/(nx+lambda))+(1-alpha^2+beta);
weightsP(2:end) = (1/(2*(nx+lambda))); 
sigmaPoints = zeros(nx,2*nx+1); 


%%


x  = x_prev + [0;0;0;0;eq(1:4)];
mes = [j1_vel;j1_ang+eq(1);j3_vel;j3_ang+eq(3);pitch_rate;pitch+eq(1)+eq(2)+eq(3);1/20;0];
Pxx = Pprev;


%%


S = chol((nx+lambda)*Pxx,'lower');
sigmaPoints(:,1) = x;
sigmaPoints(:,2:nx+1) = S(:,1:nx)+repmat(x,1,nx);
sigmaPoints(:,nx+2:2*nx+1) = -S(:,1:nx)+repmat(x,1,nx);
y_trans = mesTrans(sigmaPoints);
y_mean = y_trans*weights;
Pyy = (repmat(weightsP',8,1).*(y_trans-repmat(y_mean,1,2*nx+1)))*(y_trans-repmat(y_mean,1,2*nx+1))'+R;
Pxy = (repmat(weightsP',8,1).*(sigmaPoints-repmat(x,1,2*nx+1)))*(y_trans-repmat(y_mean,1,2*nx+1))' ;
L = Pxy/Pyy;
% mes = [j0_VEL(idx)+j1_VEL(idx);j0_ANG(idx)+j1_ANG(idx);j3_VEL(idx);j3_ANG(idx);pitch_rate(idx);1/20;0];
x = x + L*(mes-y_mean);
Pxx = Pxx - Pxy/Pyy*Pxy';


% Time update
 S = chol((nx+lambda)*Pxx,'lower');
 sigmaPoints(:,1) = x;
 sigmaPoints(:,2:nx+1) = S(:,1:nx)+repmat(x,1,nx);
 sigmaPoints(:,nx+2:2*nx+1) = -S(:,1:nx)+repmat(x,1,nx);
 x_trans = RK4(0.001,sigmaPoints,k_spring,kang,u_prev(1),u_prev(2));
 x = x_trans*weights;
 Pxx =  (repmat(weightsP',8,1).*(x_trans-repmat(x,1,2*nx+1)))*(x_trans-repmat(x,1,2*nx+1))'+Q;
 P = Pxx;



x_est = x - [0;0;0;0;eq(1:4)];




end

== matlab function simulinkControlLoop/state estimation/estimation_left ==
  data: x_prev input; x_est output; Pprev input; j1_vel input; j1_ang input; j3_vel input; j3_ang input; pitch_rate input; pitch input; u_prev input; eq input; P output; Q input; R input
function [x_est,P] = fcn(x_prev,Pprev,j1_vel,j1_ang,j3_vel,j3_ang,pitch_rate,pitch,u_prev,eq,Q,R)

x_est = zeros(8,1);
P = zeros(8,8);
k_spring = eq(5);
kang = eq(6);
nx = 8;
alpha = 1e-3;
kappa = 0;
beta = 2;
lambda = alpha^2*(nx+kappa);
weights = zeros(2*nx+1,1);
weights(1) = (lambda/(nx+lambda));
weights(2:end) = (1/(2*(nx+lambda))); 


weightsP = zeros(2*nx+1,1);
weightsP(1) = (lambda/(nx+lambda))+(1-alpha^2+beta);
weightsP(2:end) = (1/(2*(nx+lambda))); 
sigmaPoints = zeros(nx,2*nx+1); 


%%


x  = x_prev + [0;0;0;0;eq(1:4)];
mes = [j1_vel;j1_ang+eq(1);j3_vel;j3_ang+eq(3);pitch_rate;pitch+eq(1)+eq(2)+eq(3);1/20;0];
Pxx = Pprev;


%%


S = chol((nx+lambda)*Pxx,'lower');
sigmaPoints(:,1) = x;
sigmaPoints(:,2:nx+1) = S(:,1:nx)+repmat(x,1,nx);
sigmaPoints(:,nx+2:2*nx+1) = -S(:,1:nx)+repmat(x,1,nx);
y_trans = mesTrans(sigmaPoints);
y_mean = y_trans*weights;
Pyy = (repmat(weightsP',8,1).*(y_trans-repmat(y_mean,1,2*nx+1)))*(y_trans-repmat(y_mean,1,2*nx+1))'+R;
Pxy = (repmat(weightsP',8,1).*(sigmaPoints-repmat(x,1,2*nx+1)))*(y_trans-repmat(y_mean,1,2*nx+1))' ;
L = Pxy/Pyy;
% mes = [j0_VEL(idx)+j1_VEL(idx);j0_ANG(idx)+j1_ANG(idx);j3_VEL(idx);j3_ANG(idx);pitch_rate(idx);1/20;0];
x = x + L*(mes-y_mean);
Pxx = Pxx - Pxy/Pyy*Pxy';


% Time update
 S = chol((nx+lambda)*Pxx,'lower');
 sigmaPoints(:,1) = x;
 sigmaPoints(:,2:nx+1) = S(:,1:nx)+repmat(x,1,nx);
 sigmaPoints(:,nx+2:2*nx+1) = -S(:,1:nx)+repmat(x,1,nx);
 x_trans = RK4(0.001,sigmaPoints,k_spring,kang,u_prev(1),u_prev(2));
 x = x_trans*weights;
 Pxx =  (repmat(weightsP',8,1).*(x_trans-repmat(x,1,2*nx+1)))*(x_trans-repmat(x,1,2*nx+1))'+Q;
 P = Pxx;



x_est = x - [0;0;0;0;eq(1:4)];




end

== matlab function simulinkControlLoop/pendulumCTR/process_signals_L/MATLAB Function ==
  data: v3 input; th_dot3 output; th2 input; th4 input; th3 input; eq input


function th_dot3 = fcn(v3,th2,th4,th3,eq)
th2 =th2+eq(2);
th3 =th3+eq(3);
th4 =th4+eq(4);
th_dot3 =  -(193*v3.*(188*sin(th2 - th4) + 93*sin(th2 + th3 - th4)))./(17484*sin(th3));

== matlab function simulinkControlLoop/pendulumCTR/procces_signals_R/MATLAB Function1 ==
  data: v3 input; th_dot3 output; th2 input; th4 input; th3 input; eq input; dth1 input; pitch_rate output


function [th_dot3,pitch_rate] = fcn(v3,th2,th4,th3,eq,dth1)
th2 =th2+eq(2);
th3 =th3+eq(3);
th4 =th4+eq(4);
th_dot3 =  -(193*v3.*(188*sin(th2 - th4) + 93*sin(th2 + th3 - th4)))./(17484*sin(th3));
th_dot2 = (193*v3*sin(th2 + th3 - th4))/(188*sin(th3));
pitch_rate = th_dot2 +th_dot3 + dth1;
